simulink model "systema"  (Simulink 8.3)
settings: Solver=ode3  StartTime=0.0  StopTime=200  FixedStep=0.01  RelTol=1e-3
InitFcn:
  | Model.modelsiminit
StartFcn:
  | Model.modelsiminit
libraries: simulink x10
CloseFcn:
  | rtwprivate ssgencode ModelCloseRequest systema
settings Model: Creator=Keshav Sarraf  LastModifiedBy=keshav  BufferReuse=off
settings DataIOCC: SignalLoggingName=sigsOut
settings OptimizationCC: OptimizeBlockIOStorage=off  BufferReuse=off  GlobalBufferReuse=off  ExpressionFolding=off  FoldNonRolledExpr=off  LocalBlockOutputs=off  InitFltsAndDblsToZero=on
settings DebuggingCC: SaveWithParameterizedLinksMsg=none  SignalResolutionControl=TryResolveAllWithWarning  SolverPrmCheckMsg=none  MultiTaskDSMMsg=warning  MultiTaskCondExecSysMsg=none  FcnCallInpInsideContextMsg=UseLocalSettings
settings HardwareCC: TargetUnknown=on
settings SFSimCC: SimParseCustomCode=off
settings RTWCC: IncludeERTFirstTime=on
settings CodeAppCC: IgnoreCustomStorageClasses=off
settings GRTTargetCC: TargetFcnLib=ansi_tfl_tmw.mat  ModelReferenceCompliant=off  MatFileLogging=off

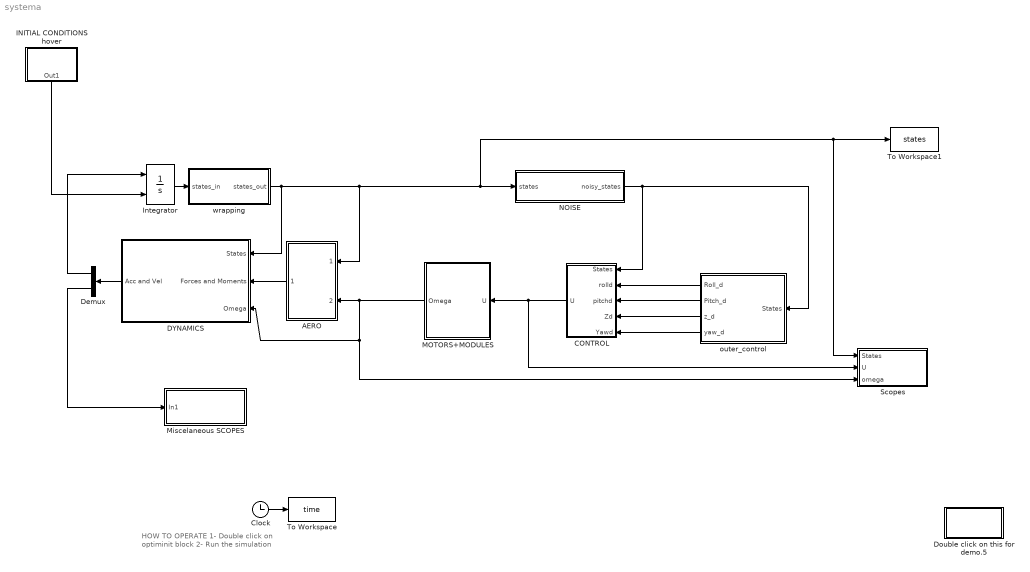
== system systema ==
  note: HOW TO OPERATE
      | 1- Double click on optiminit block
      | 2- Run the simulation
  AERO : Subsystem
  CONTROL : Subsystem
  Clock : Clock
  DYNAMICS : Subsystem
  Demux : Demux  Outputs=2
  Double click on this for demo.5 : Subsystem
      settings: OpenFcn=optsiminit
      mask Display: disp('optsiminit')
  INITIAL CONDITIONS hover : Subsystem
  Integrator : Integrator  InitialConditionSource=external
  MOTORS+MODULES : Subsystem
  Miscelaneous SCOPES : Subsystem
  "NOISE " : Subsystem
  Scopes : Subsystem
  To Workspace : ToWorkspace  VariableName=time  SampleTime=-1
  To Workspace1 : ToWorkspace  VariableName=states  SaveFormat=Structure With Time  SampleTime=-1
  outer_control : Subsystem
  wrapping : Subsystem
  wires:
  Clock/1 -> To Workspace/1
  DYNAMICS/1(Acc and Vel) -> Demux/1
  Demux/1 -> Integrator/1
  Demux/2 -> Miscelaneous SCOPES/1(In1)
  CONTROL/1(U) -> Scopes/2(U), MOTORS+MODULES/1(U)
  MOTORS+MODULES/1(Omega) -> Scopes/3(omega), DYNAMICS/3(Omega), AERO/2(Omega)
  AERO/1(F & M) -> DYNAMICS/2(Forces and Moments)
  Integrator/1 -> wrapping/1(states_in)
  "NOISE "/1(noisy_states) -> CONTROL/1(States), outer_control/1(States)
  outer_control/3(z_d) -> CONTROL/4(Zd)
  outer_control/4(yaw_d) -> CONTROL/5(Yawd)
  outer_control/2(Pitch_d) -> CONTROL/3(pitchd)
  outer_control/1(Roll_d) -> CONTROL/2(rolld)
  wrapping/1(states_out) -> AERO/1(States), "NOISE "/1(states), To Workspace1/1, Scopes/1(States), DYNAMICS/1(States)
  INITIAL CONDITIONS hover/1(Out1) -> Integrator/2

== system systema/AERO ==
  note: Forces and
      | Moments
  States : Inport
  Omega : Inport  Port=2
  AERO Attitude [rad] : MATLABFcn  MATLABFcn=Model.aero  OutputDimensions=24
  Mux1 : Mux  Inputs=3
  Step : Step  Time=30  Before=4  After=4  SampleTime=0
  F & M : Outport
  wires:
  States/1 -> Mux1/1
  Omega/1 -> Mux1/2
  Mux1/1 -> AERO Attitude [rad]/1
  AERO Attitude [rad]/1 -> F & M/1
  Step/1 -> Mux1/3

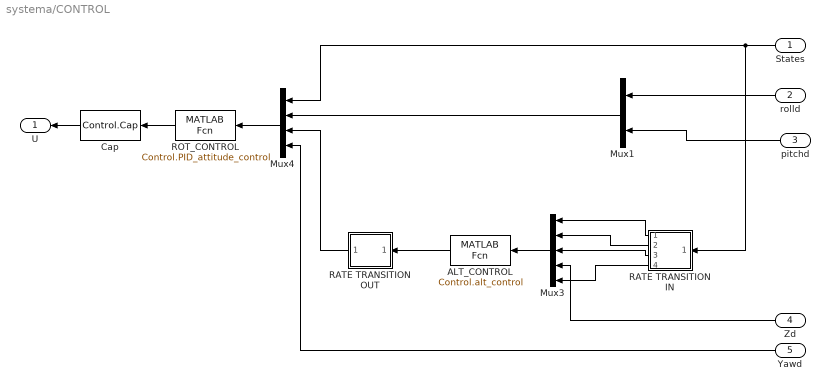
== system systema/CONTROL ==
  States : Inport
  rolld : Inport  Port=2
  pitchd : Inport  Port=3
  Zd : Inport  Port=4
  Yawd : Inport  Port=5
  ALT_CONTROL : MATLABFcn  MATLABFcn=Control.alt_control  OutputDimensions=1  SampleTime=0.05
  Cap : MATLABFcn  MATLABFcn=Control.Cap  OutputDimensions=4  OutputSignalType=real
  Mux1 : Mux  Inputs=2
  Mux3 : Mux  Inputs=5
  Mux4 : Mux
  RATE TRANSITION IN : Subsystem
  RATE TRANSITION OUT : Subsystem
  ROT_CONTROL : MATLABFcn  MATLABFcn=Control.PID_attitude_control  OutputDimensions=4
  U : Outport
  wires:
  pitchd/1 -> Mux1/2
  rolld/1 -> Mux1/1
  Zd/1 -> Mux3/4
  RATE TRANSITION IN/3(Out3) -> Mux3/3
  RATE TRANSITION IN/2(Out2) -> Mux3/2
  RATE TRANSITION IN/1(Out1) -> Mux3/1
  Mux3/1 -> ALT_CONTROL/1
  RATE TRANSITION OUT/1(Out1) -> Mux4/3
  Yawd/1 -> Mux4/4
  ALT_CONTROL/1 -> RATE TRANSITION OUT/1(In1)
  Mux4/1 -> ROT_CONTROL/1
  Mux1/1 -> Mux4/2
  States/1 -> RATE TRANSITION IN/1(In1), Mux4/1
  ROT_CONTROL/1 -> Cap/1
  Cap/1 -> U/1
  RATE TRANSITION IN/4(Out4) -> Mux3/5

== system systema/DYNAMICS ==
  States : Inport
  Forces and Moments : Inport  Port=2
  Omega : Inport  Port=3
  DYNAMICS : MATLABFcn  MATLABFcn=Model.dinamica  OutputDimensions=18
  Mux1 : Mux  Inputs=3
  Acc and Vel : Outport
  wires:
  DYNAMICS/1 -> Acc and Vel/1
  Mux1/1 -> DYNAMICS/1
  Forces and Moments/1 -> Mux1/2
  States/1 -> Mux1/1
  Omega/1 -> Mux1/3

== system systema/Double click on this for demo.5 ==

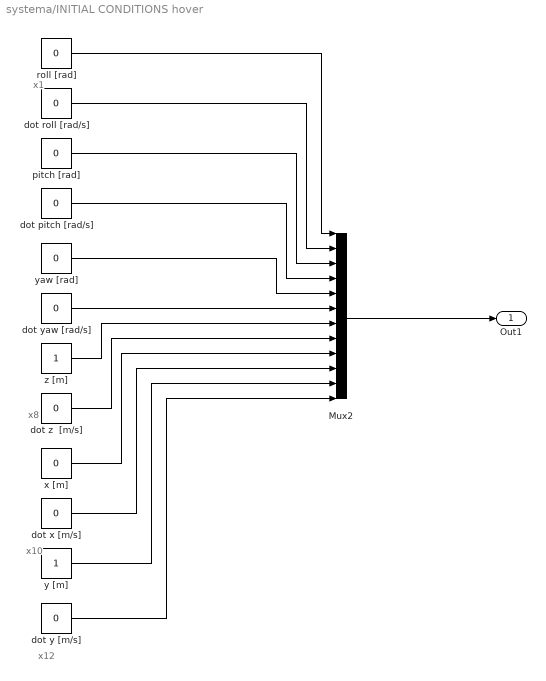
== system systema/INITIAL CONDITIONS hover ==
  note: x8
  note: x10
  note: x12
  note: x1
  Mux2 : Mux  Inputs=12
  dot pitch [rad/s] : Constant  Value=0
  dot roll [rad/s] : Constant  Value=0
  dot x [m/s] : Constant  Value=0
  dot y [m/s] : Constant  Value=0
  dot yaw [rad/s] : Constant  Value=0
  dot z  [m/s] : Constant  Value=0
  pitch [rad] : Constant  Value=0
  roll [rad] : Constant  Value=0
  x [m] : Constant  Value=0
  y [m] : Constant
  yaw [rad] : Constant  Value=0
  z [m] : Constant
  Out1 : Outport
  wires:
  dot y [m/s]/1 -> Mux2/12
  y [m]/1 -> Mux2/11
  dot x [m/s]/1 -> Mux2/10
  x [m]/1 -> Mux2/9
  Mux2/1 -> Out1/1
  yaw [rad]/1 -> Mux2/5
  dot z  [m/s]/1 -> Mux2/8
  z [m]/1 -> Mux2/7
  dot yaw [rad/s]/1 -> Mux2/6
  dot pitch [rad/s]/1 -> Mux2/4
  pitch [rad]/1 -> Mux2/3
  dot roll [rad/s]/1 -> Mux2/2
  roll [rad]/1 -> Mux2/1

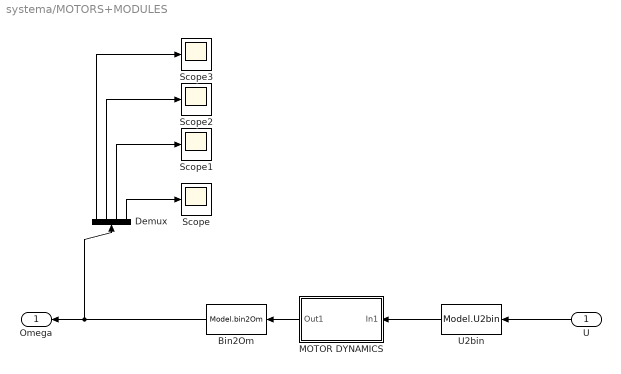
== system systema/MOTORS+MODULES ==
  U : Inport
  Bin2Om : MATLABFcn  MATLABFcn=Model.bin2Om  OutputDimensions=4  OutputSignalType=real
  Demux : Demux
  MOTOR DYNAMICS : Subsystem
  Scope{,1..3} (4 alike) : Scope
      Scope settings: SaveName=ScopeData27
      Scope1 settings: SaveName=ScopeData41
      Scope2 settings: SaveName=ScopeData42
      Scope3 settings: SaveName=ScopeData43
  U2bin : MATLABFcn  MATLABFcn=Model.U2bin  OutputDimensions=4  OutputSignalType=real
  Omega : Outport
  wires:
  MOTOR DYNAMICS/1(Out1) -> Bin2Om/1
  U2bin/1 -> MOTOR DYNAMICS/1(In1)
  U/1 -> U2bin/1
  Demux/4 -> Scope/1
  Demux/3 -> Scope1/1
  Demux/2 -> Scope2/1
  Demux/1 -> Scope3/1
  Bin2Om/1 -> Demux/1, Omega/1

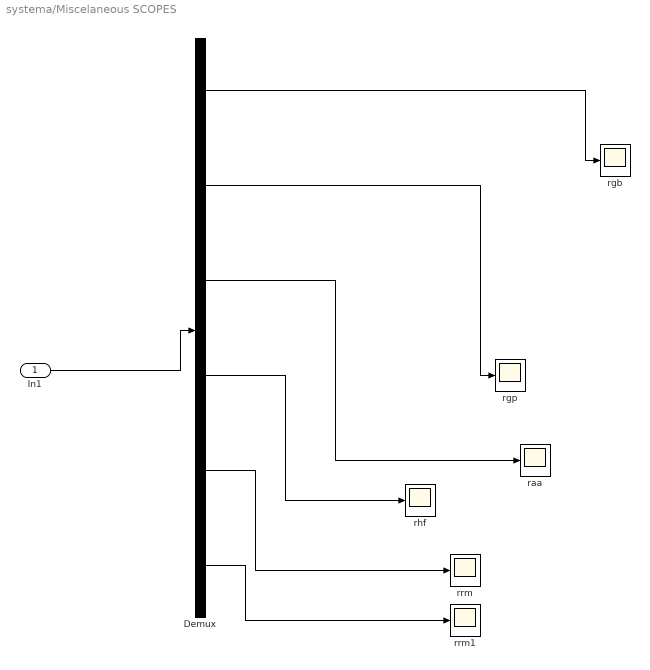
== system systema/Miscelaneous SCOPES ==
  In1 : Inport  PortDimensions=6
  Demux : Demux  Outputs=6
  raa : Scope
      settings: TimeRange=18  YMin=-200  YMax=200  SaveName=ScopeData16
  rgb : Scope
      settings: YMin=-0.25  YMax=-0.05  SaveName=ScopeData14
  rgp : Scope
      settings: YMin=-2250  YMax=2250  SaveName=ScopeData15
  rhf : Scope
      settings: TimeRange=10  YMin=-110.5  YMax=-107.25  SaveName=ScopeData18
  rrm : Scope
      settings: TimeRange=5  YMin=-4.75e-015  YMax=0  SaveName=ScopeData25
  rrm1 : Scope
      settings: TimeRange=5  YMin=-4.75e-015  YMax=0  SaveName=ScopeData3
  wires:
  In1/1 -> Demux/1
  Demux/5 -> rrm/1
  Demux/4 -> rhf/1
  Demux/3 -> raa/1
  Demux/2 -> rgp/1
  Demux/1 -> rgb/1
  Demux/6 -> rrm1/1

== system systema/NOISE  ==
  states : Inport
  NOISY DATA SCOPES Attitude [rad] Ang. rates [rad/sec] position [m] Pos. rates [m/s]1 : Subsystem
  W. NORMAL NOISE : Subsystem
  noisy_states : Outport
  wires:
  states/1 -> W. NORMAL NOISE/1(In1)
  W. NORMAL NOISE/1(Out1) -> noisy_states/1, NOISY DATA SCOPES Attitude [rad] Ang. rates [rad/sec] position [m] Pos. rates [m/s]1/1(In1)

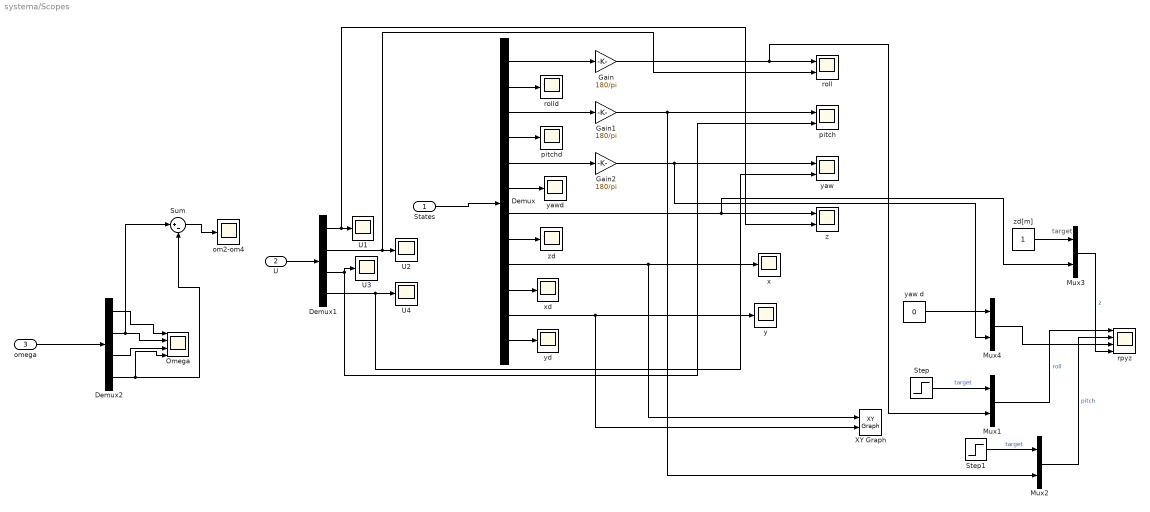
== system systema/Scopes ==
  note: target
  States : Inport
  U : Inport  Port=2
  omega : Inport  Port=3
  Demux : Demux  Outputs=12
  Demux1 : Demux
  Demux2 : Demux
  Gain : Gain  Gain=180/pi
  Gain1 : Gain  Gain=180/pi
  Gain2 : Gain  Gain=180/pi
  Mux{1..4} (4 alike) : Mux  Inputs=2
  Omega : Scope  NumInputPorts=4
      settings: TimeRange=3.5  YMin=299.78~127.77~298.75~132.05  YMax=299.91~127.835~300.5~132.6  SaveName=ScopeData11
  Step : Step  Time=10  After=0  SampleTime=0
  Step1 : Step  Time=20  After=0  SampleTime=0
  Sum : Sum  Inputs=|+-
  U{1..4} (4 alike) : Scope
      U1 settings: TimeRange=3.5  YMin=144.101  YMax=144.104  SaveName=ScopeData36
      U2 settings: YMin=142.5  YMax=147.5  SaveName=ScopeData37
      U3 settings: YMin=0  YMax=150  SaveName=ScopeData38
      U4 settings: YMin=0  YMax=150  SaveName=ScopeData39
  XY Graph : simulink/Sinks/XY Graph  xmin=-3  xmax=3  ymin=-3  ymax=3  st=-1
  om2-om4 : Scope
      settings: TimeRange=40  YMin=-2  YMax=14  SaveName=ScopeData40
  pitch : Scope  NumInputPorts=2
      settings: TimeRange=4  YMin=7.5~-5  YMax=11.75~5  SaveName=ScopeData13
  pitchd : Scope
      settings: YMin=-1.75  YMax=1.75  SaveName=ScopeData21
  roll : Scope  NumInputPorts=2
      settings: TimeRange=35  YMin=-1~-15  YMax=12~25  SaveName=ScopeData22
  rolld : Scope
      settings: TimeRange=7  YMin=-0.15  YMax=0.125  SaveName=ScopeData23
  rpyz : Scope  NumInputPorts=4
      settings: TimeRange=100  YMin=-30~-15~-2.5~0.5  YMax=60~25~17.5~4.5  SaveName=ScopeData12
  x : Scope
      settings: TimeRange=5  YMin=-15  YMax=35  SaveName=ScopeData28
  xd : Scope
      settings: TimeRange=5  YMin=-1.5  YMax=2.25  SaveName=ScopeData29
  y : Scope
      settings: TimeRange=5  YMin=0.964  YMax=0.988  SaveName=ScopeData30
  yaw : Scope  NumInputPorts=2
      settings: TimeRange=5  YMin=-1.75~-0.1  YMax=1~1  SaveName=ScopeData31
  yaw d : Constant  Value=0
  yawd : Scope
      settings: TimeRange=18  YMin=-0.275  YMax=0.15  SaveName=ScopeData32
  yd : Scope
      settings: TimeRange=5  YMin=-143.75  YMax=-141.75  SaveName=ScopeData33
  z : Scope  NumInputPorts=2
      settings: TimeRange=40  YMin=0.55~0  YMax=5~50  SaveName=ScopeData34
  zd : Scope
      settings: TimeRange=10  YMin=-2  YMax=2  SaveName=ScopeData35
  zd[m] : Constant
  wires:
  Demux/3 -> Gain1/1
  Demux/5 -> Gain2/1
  Demux/2 -> rolld/1
  Demux/6 -> yawd/1
  Demux/7 -> Mux3/2, z/1
  Demux/8 -> zd/1
  Demux/9 -> XY Graph/1, x/1
  Demux/11 -> XY Graph/2, y/1
  Demux/12 -> yd/1
  Demux/10 -> xd/1
  Demux/4 -> pitchd/1
  Demux/1 -> Gain/1
  States/1 -> Demux/1
  Demux1/1 -> z/2, U1/1
  Demux1/3 -> pitch/2, U3/1
  Demux1/4 -> yaw/2, U4/1
  U/1 -> Demux1/1
  Demux1/2 -> roll/2, U2/1
  omega/1 -> Demux2/1
  Gain/1 -> Mux1/2, roll/1
  Gain1/1 -> Mux2/2, pitch/1
  Gain2/1 -> Mux4/2, yaw/1
  Demux2/1 -> Omega/1
  Demux2/2 -> Sum/1, Omega/2
  Demux2/3 -> Omega/3
  Demux2/4 -> Sum/2, Omega/4
  Sum/1 -> om2-om4/1
  Step/1 -> Mux1/1  "target"
  Step1/1 -> Mux2/1  "target"
  Mux1/1 -> rpyz/1  "roll"
  Mux2/1 -> rpyz/2  "pitch"
  zd[m]/1 -> Mux3/1
  Mux3/1 -> rpyz/4  "z"
  Mux4/1 -> rpyz/3
  yaw d/1 -> Mux4/1

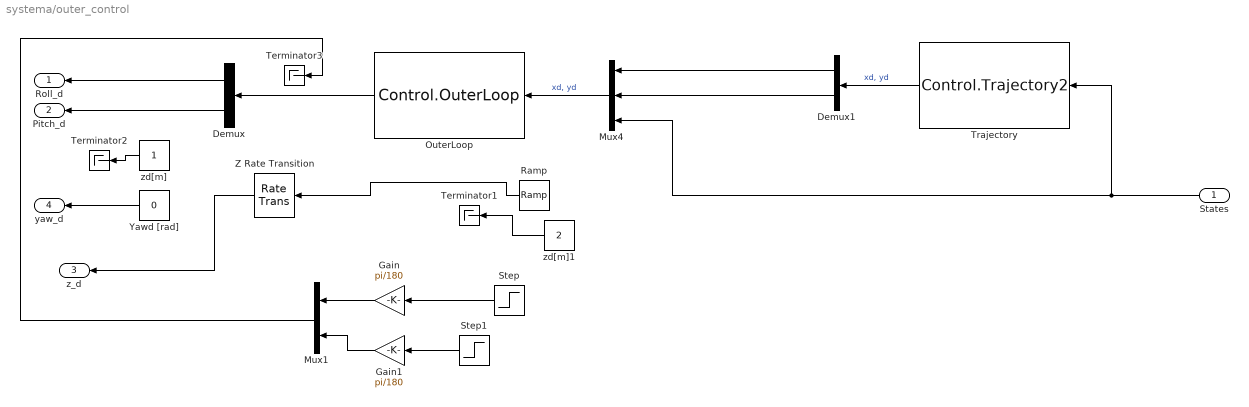
== system systema/outer_control ==
  States : Inport
  Demux : Demux  Outputs=2
  Demux1 : Demux  Outputs=2
  Gain : Gain  Gain=pi/180
  Gain1 : Gain  Gain=pi/180
  Mux1 : Mux  Inputs=2
  Mux4 : Mux  Inputs=3
  OuterLoop : MATLABFcn  MATLABFcn=Control.OuterLoop  OutputDimensions=2
  Ramp : simulink/Sources/Ramp  slope=2/200  start=0  X0=1
  Step : Step  Time=0  SampleTime=0
  Step1 : Step  Time=10  After=0  SampleTime=0
  Terminator1 : Terminator
  Terminator2 : Terminator
  Terminator3 : Terminator
  Trajectory : MATLABFcn  MATLABFcn=Control.Trajectory2  OutputDimensions=2
  Yawd [rad] : Constant  Value=0
  Z Rate Transition : RateTransition  Deterministic=off  OutPortSampleTime=50E-3
  zd[m] : Constant
  zd[m]1 : Constant  Value=2
  Roll_d : Outport
  Pitch_d : Outport  Port=2
  z_d : Outport  Port=3
  yaw_d : Outport  Port=4
  wires:
  Step/1 -> Gain/1
  Yawd [rad]/1 -> yaw_d/1
  Step1/1 -> Gain1/1
  States/1 -> Trajectory/1, Mux4/3
  Mux4/1 -> OuterLoop/1  "xd, yd"
  Demux/2 -> Pitch_d/1
  Demux/1 -> Roll_d/1
  Trajectory/1 -> Demux1/1  "xd, yd"
  Gain/1 -> Mux1/1
  Gain1/1 -> Mux1/2
  Z Rate Transition/1 -> z_d/1
  zd[m]/1 -> Terminator2/1
  OuterLoop/1 -> Demux/1
  Mux1/1 -> Terminator3/1
  Demux1/2 -> Mux4/2
  Demux1/1 -> Mux4/1
  zd[m]1/1 -> Terminator1/1
  Ramp/1 -> Z Rate Transition/1

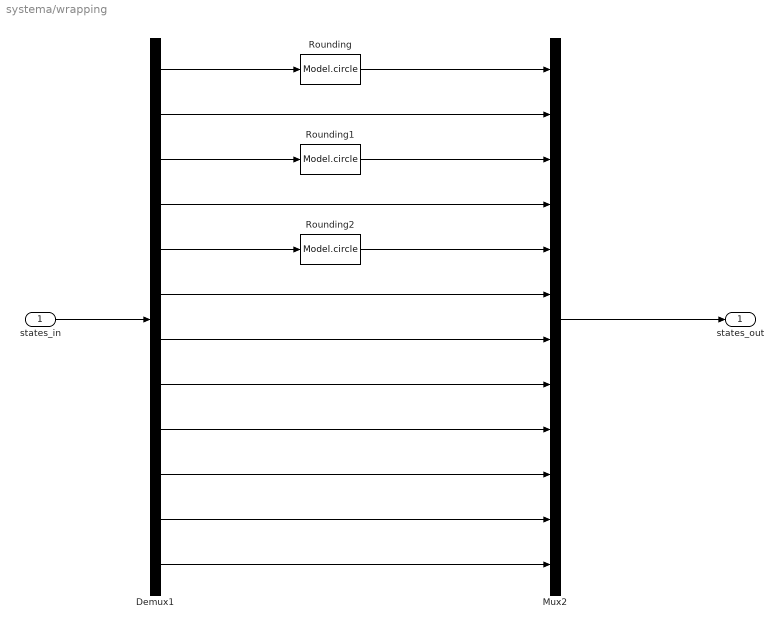
== system systema/wrapping ==
  states_in : Inport
  Demux1 : Demux  Outputs=12
  Mux2 : Mux  Inputs=12
  Rounding : MATLABFcn  MATLABFcn=Model.circle  OutputDimensions=1
  Rounding1 : MATLABFcn  MATLABFcn=Model.circle  OutputDimensions=1
  Rounding2 : MATLABFcn  MATLABFcn=Model.circle  OutputDimensions=1
  states_out : Outport
  wires:
  Demux1/11 -> Mux2/11
  Demux1/6 -> Mux2/6
  Demux1/10 -> Mux2/10
  Demux1/8 -> Mux2/8
  Demux1/5 -> Rounding2/1
  Demux1/12 -> Mux2/12
  Demux1/9 -> Mux2/9
  Demux1/7 -> Mux2/7
  Demux1/3 -> Rounding1/1
  Demux1/4 -> Mux2/4
  Demux1/2 -> Mux2/2
  Demux1/1 -> Rounding/1
  states_in/1 -> Demux1/1
  Mux2/1 -> states_out/1
  Rounding/1 -> Mux2/1
  Rounding1/1 -> Mux2/3
  Rounding2/1 -> Mux2/5

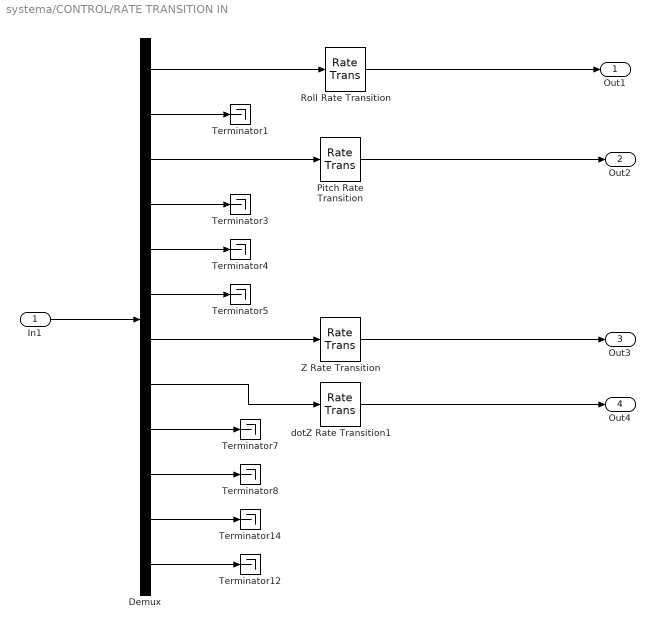
== system systema/CONTROL/RATE TRANSITION IN ==
  In1 : Inport
  Demux : Demux  Outputs=12
  Pitch Rate Transition : RateTransition  Deterministic=off  OutPortSampleTime=50E-3
  Roll Rate Transition : RateTransition  Deterministic=off  OutPortSampleTime=50E-3
  Terminator{1,3..5,7..8,12,14} (8 alike) : Terminator
  Z Rate Transition : RateTransition  Deterministic=off  OutPortSampleTime=50E-3
  dotZ Rate Transition1 : RateTransition  Deterministic=off  OutPortSampleTime=50E-3
  Out1 : Outport
  Out2 : Outport  Port=2
  Out3 : Outport  Port=3
  Out4 : Outport  Port=4
  wires:
  Z Rate Transition/1 -> Out3/1
  Pitch Rate Transition/1 -> Out2/1
  Roll Rate Transition/1 -> Out1/1
  Demux/8 -> dotZ Rate Transition1/1
  Demux/12 -> Terminator12/1
  Demux/11 -> Terminator14/1
  Demux/10 -> Terminator8/1
  Demux/9 -> Terminator7/1
  Demux/6 -> Terminator5/1
  Demux/5 -> Terminator4/1
  Demux/4 -> Terminator3/1
  Demux/3 -> Pitch Rate Transition/1
  Demux/2 -> Terminator1/1
  Demux/1 -> Roll Rate Transition/1
  In1/1 -> Demux/1
  Demux/7 -> Z Rate Transition/1
  dotZ Rate Transition1/1 -> Out4/1

== system systema/CONTROL/RATE TRANSITION OUT ==
  In1 : Inport
  Rate Transition1 : RateTransition  Deterministic=off
  Out1 : Outport
  wires:
  Rate Transition1/1 -> Out1/1
  In1/1 -> Rate Transition1/1

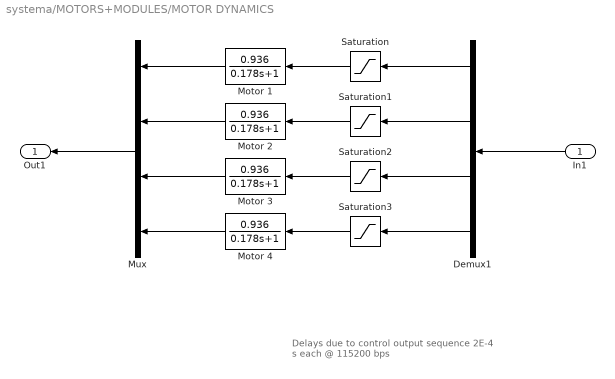
== system systema/MOTORS+MODULES/MOTOR DYNAMICS ==
  note: Delays due to control output sequence
      | 2E-4 s each @ 115200 bps
  In1 : Inport
  Demux1 : Demux
  Motor {1..4} (4 alike) : TransferFcn  Numerator=[0.936]  Denominator=[0.178 1]
  Mux : Mux
  Saturation{,1..3} (4 alike) : Saturate  UpperLimit=250  LowerLimit=0
  Out1 : Outport
  wires:
  In1/1 -> Demux1/1
  Demux1/1 -> Saturation/1
  Demux1/2 -> Saturation1/1
  Demux1/3 -> Saturation2/1
  Demux1/4 -> Saturation3/1
  Mux/1 -> Out1/1
  Motor 2/1 -> Mux/2
  Motor 3/1 -> Mux/3
  Motor 4/1 -> Mux/4
  Motor 1/1 -> Mux/1
  Saturation/1 -> Motor 1/1
  Saturation1/1 -> Motor 2/1
  Saturation2/1 -> Motor 3/1
  Saturation3/1 -> Motor 4/1

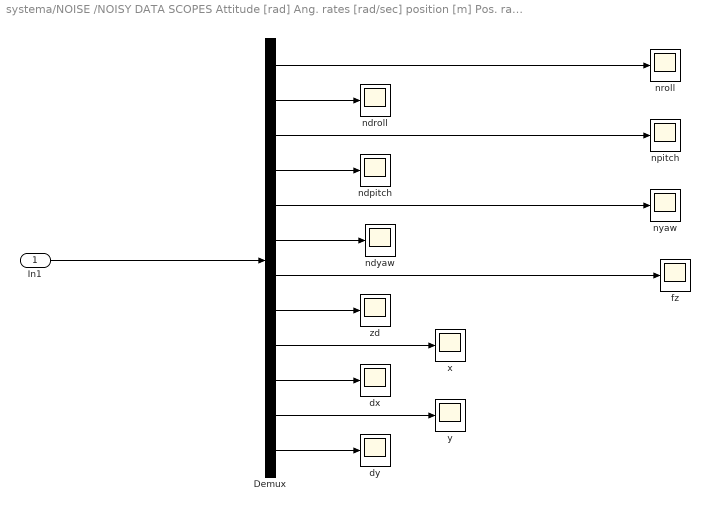
== system systema/NOISE /NOISY DATA SCOPES Attitude [rad] Ang. rates [rad/sec] position [m] Pos. rates [m/s]1 ==
  In1 : Inport
  Demux : Demux  Outputs=12
  dx : Scope
      settings: TimeRange=5  YMin=0  YMax=0.009  SaveName=ScopeData5
  dy : Scope
      settings: TimeRange=5  YMin=0  YMax=0.009  SaveName=ScopeData10
  fz : Scope
      settings: TimeRange=5  YMin=0  YMax=0.009  SaveName=ScopeData17
  ndpitch : Scope
      settings: YMin=-2250  YMax=2250  SaveName=ScopeData15
  ndroll : Scope
      settings: YMin=-0.25  YMax=-0.05  SaveName=ScopeData14
  ndyaw : Scope
      settings: TimeRange=18  YMin=-200  YMax=200  SaveName=ScopeData16
  npitch : Scope
      settings: TimeRange=4  YMin=-1  YMax=1
  nroll : Scope
      settings: TimeRange=60  YMin=-0.1  YMax=0.45
  nyaw : Scope
      settings: TimeRange=5  YMin=0  YMax=0.22  SaveName=ScopeData2
  x : Scope
      settings: TimeRange=5  YMin=0  YMax=0.009  SaveName=ScopeData4
  y : Scope
      settings: TimeRange=5  YMin=0  YMax=0.009  SaveName=ScopeData6
  zd : Scope
      settings: TimeRange=10  YMin=-110.5  YMax=-107.25  SaveName=ScopeData18
  wires:
  Demux/1 -> nroll/1
  Demux/4 -> ndpitch/1
  Demux/8 -> zd/1
  Demux/7 -> fz/1
  Demux/6 -> ndyaw/1
  Demux/2 -> ndroll/1
  Demux/5 -> nyaw/1
  Demux/3 -> npitch/1
  In1/1 -> Demux/1
  Demux/9 -> x/1
  Demux/10 -> dx/1
  Demux/11 -> y/1
  Demux/12 -> dy/1

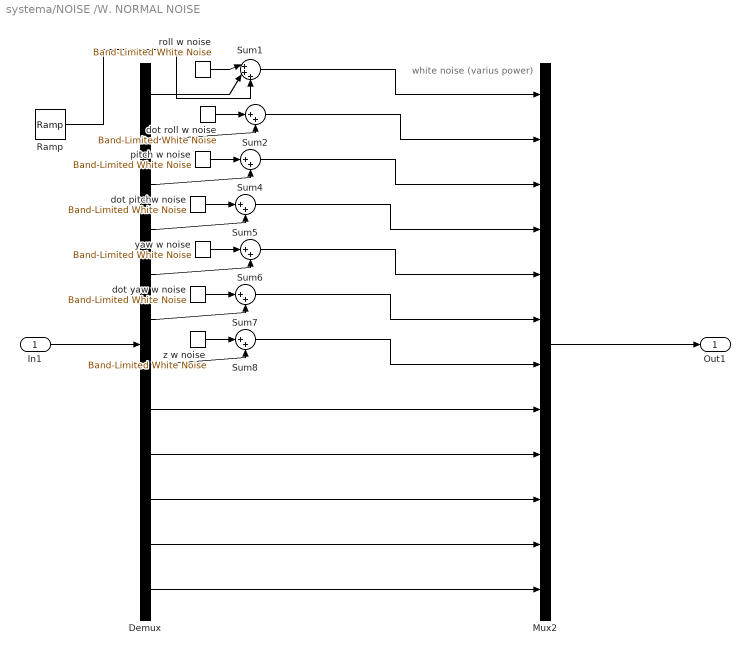
== system systema/NOISE /W. NORMAL NOISE ==
  note: white noise (varius power)
  In1 : Inport
  Demux : Demux  Outputs=12
  Mux2 : Mux  Inputs=12
  Ramp : simulink/Sources/Ramp  slope=0  start=20  X0=0
  Sum1 : Sum  Inputs=|+++  SaturateOnIntegerOverflow=on
  Sum{2,4..8} (6 alike) : Sum  Inputs=|++  SaturateOnIntegerOverflow=on
  dot pitchw noise : simulink/Sources/Band-Limited White Noise  Cov=[0.0001]  Ts=0.01  seed=[23341]
  dot roll w noise : simulink/Sources/Band-Limited White Noise  Cov=[0.0001]  Ts=0.01  seed=[23341]
  dot yaw w noise : simulink/Sources/Band-Limited White Noise  Cov=[0.0001]  Ts=0.01  seed=[23341]
  pitch w noise : simulink/Sources/Band-Limited White Noise  Cov=[0.00001]  Ts=0.01  seed=[23341]
  roll w noise : simulink/Sources/Band-Limited White Noise  Cov=[0.000001]  Ts=0.01  seed=[24431]
  yaw w noise : simulink/Sources/Band-Limited White Noise  Cov=[0.00001]  Ts=0.01  seed=[23341]
  z w noise : simulink/Sources/Band-Limited White Noise  Cov=[0.00001]  Ts=0.01  seed=[23341]
  Out1 : Outport
  wires:
  Demux/8 -> Mux2/8
  Demux/12 -> Mux2/12
  Demux/11 -> Mux2/11
  Demux/10 -> Mux2/10
  Demux/9 -> Mux2/9
  Sum8/1 -> Mux2/7
  z w noise/1 -> Sum8/1
  Demux/7 -> Sum8/2
  Sum7/1 -> Mux2/6
  dot yaw w noise/1 -> Sum7/1
  Demux/6 -> Sum7/2
  Sum6/1 -> Mux2/5
  yaw w noise/1 -> Sum6/1
  Demux/5 -> Sum6/2
  Sum5/1 -> Mux2/4
  dot pitchw noise/1 -> Sum5/1
  Demux/4 -> Sum5/2
  Sum4/1 -> Mux2/3
  pitch w noise/1 -> Sum4/1
  Demux/3 -> Sum4/2
  Sum2/1 -> Mux2/2
  dot roll w noise/1 -> Sum2/1
  Demux/2 -> Sum2/2
  Sum1/1 -> Mux2/1
  roll w noise/1 -> Sum1/1
  Mux2/1 -> Out1/1
  In1/1 -> Demux/1
  Demux/1 -> Sum1/2
  Ramp/1 -> Sum1/3
